simulink model "x244"  (R2018b)
settings: Solver=VariableStepAuto  StartTime=0.0  StopTime=10.0  RelTol=1e-3
PostLoadFcn:
  | if any(exist('dsrtsu_mdlpostloadfcn', 'file') ~= 0), dsrtsu_mdlpostloadfcn('Execute', bdroot); end
libraries: simulink x1
settings Model: DSRTSU_INTERNAL_RTI_VER=540  DSRTSU_INTERNAL_RTI_TYPE=rti1401  Creator=Administrator  LastModifiedBy=Administrator

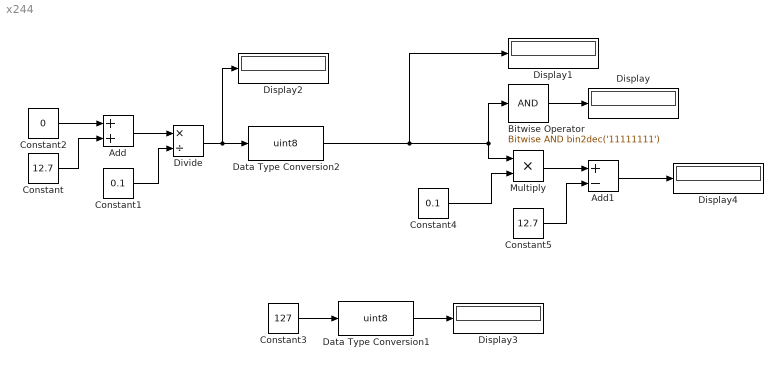
== system x244 ==
  Add : Sum
  Add1 : Sum  Inputs=+-
  Bitwise Operator : simulink/Logic and Bit Operations/Bitwise Operator  logicop=AND  UseBitMask=on  BitMask=bin2dec('11111111')  BitMaskRealWorld=Stored Integer
  Constant : Constant  Value=12.7
  Constant1 : Constant  Value=0.1
  Constant2 : Constant  Value=0  OutDataTypeStr=single
  Constant3 : Constant  Value=127
  Constant4 : Constant  Value=0.1
  Constant5 : Constant  Value=12.7
  Data Type Conversion1 : DataTypeConversion  OutDataTypeStr=uint8
  Data Type Conversion2 : DataTypeConversion  OutDataTypeStr=uint8
  Display{,1..4} (5 alike) : Display
      Display settings: Format=hex (Stored Integer)
      Display1 settings: Format=binary (Stored Integer)
      Display2 settings: Format=binary (Stored Integer)
      Display3 settings: Format=hex (Stored Integer)
  Divide : Product  Inputs=*/  OutDataTypeStr=single
  Multiply : Product
  wires:
  Multiply/1 -> Add1/1
  Constant1/1 -> Divide/2
  Add/1 -> Divide/1
  Constant5/1 -> Add1/2
  Divide/1 -> Display2/1, Data Type Conversion2/1
  Constant/1 -> Add/2
  Data Type Conversion2/1 -> Display1/1, Multiply/1, Bitwise Operator/1
  Constant4/1 -> Multiply/2
  Constant2/1 -> Add/1
  Bitwise Operator/1 -> Display/1
  Constant3/1 -> Data Type Conversion1/1
  Data Type Conversion1/1 -> Display3/1
  Add1/1 -> Display4/1
